simulink model "S250205simul_switch_2023a"  (R2024b)
settings: Solver=FixedStepDiscrete  StartTime=0  StopTime=60  FixedStep=0.01  RelTol=1e-3  AbsTol=1e-6
undefined symbols (not defined in the file or in its folder): a, b, c, d, f, g, switch_logic, VmcRgn_C_C, VmcRgn_J_C, VmcRgn_k_1to2_C, VmcRgn_k_2to3_C, VmcRgn_k_2to6_C, VmcRgn_k_3to4_C, VmcRgn_k_5to2_C, VmcRgn_k_6to2_C, VmcRgn_Kp_C, VmcRgn_L_C, VmcRgn_lf_C, VmcRgn_lr_C, VmcRgn_mass_C, VmcRgn_Mot2Whl_C, VmcRgn_PedDep_thrs_C, VmcRgn_phs2_k_C, VmcRgn_phs2_tq_C, VmcRgn_phs3_tq_C, VmcRgn_phs4_tq_C, VmcRgn_phs5_tq_C, VmcRgn_phs6_tq_C, VmcRgn_r_e_C, VmcRgn_R_whl_C, VmcRgn_SAS_thrs_C, VmcRgn_slip_max_C, VmcRgn_slip_max_gain_F_C, VmcRgn_slip_max_gain_R_C, VmcRgn_sup_tq_C, VmcRgn_t_pred_C, VmcRgn_target_w_acc_C, VmcRgn_tTs, VmcRgn_tTsinMs_C, VmcRgn_Yaw_thrs_C, yaw_flag
libraries: simulink x26, simulink_need_slupdate x1
(part 1 of 3)
settings Model: Creator=jhu  LastModifiedBy=jshan
settings SolverCC: AutoScaleAbsTol=off
settings DataIOCC: SaveFormat=Array  SignalLoggingSaveFormat=ModelDataLogs  ReturnWorkspaceOutputs=off  SignalLoggingName=sigsOut
settings OptimizationCC: BlockReduction=off  BooleanDataType=off  ExpressionDepthLimit=2147483647  LifeSpan=inf
settings DebuggingCC: SaveWithParameterizedLinksMsg=none  UnderspecifiedInitializationDetection=Classic  MergeDetectMultiDrivingBlocksExec=none  SignalResolutionControl=TryResolveAllWithWarning  MultiTaskDSMMsg=warning  MultiTaskCondExecSysMsg=none  FcnCallInpInsideContextMsg=warning  UnconnectedInputMsg=warning  UnconnectedOutputMsg=warning  UnconnectedLineMsg=warning  StateNameClashWarn=warning  SFUnexpectedBacktrackingDiag=warning  SFNoUnconditionalDefaultTransitionDiag=warning  SFExecutionAtInitializationDiag=none  ArithmeticOperatorsInVariantConditions=warning
settings HardwareCC: ProdBitPerPointer=32  ProdBitPerSizeT=32  ProdBitPerPtrDiffT=32  ProdLargestAtomicFloat=None  ProdIntDivRoundTo=Undefined  ProdEndianess=Unspecified  ProdWordSize=32  ProdHWDeviceType=32-bit Generic  TargetUnknown=on
settings ModelReferenceCC: PropagateSignalLabelsOutOfModel=off
settings SFSimCC: SimUseLocalCustomCode=off  CustomCodeUndefinedFunction=UseInterfaceOnly
settings RTWCC: TemplateMakefile=grt_vc.tmf  RTWUseLocalCustomCode=off  GPUComputeCapability=3.5
settings CodeAppCC: StateflowObjectComments=on
settings GRTTargetCC: TargetFcnLib=ansi_tfl_tmw.mat  TargetLangStandard=C89/C90 (ANSI)  CombineOutputUpdateFcns=off  GRTInterface=on
settings ConfigComp: CovMetricSettings=dw  CovSaveCumulativeToWorkspaceVar=on  CovSaveSingleToWorkspaceVar=on  CovExternalEMLEnable=off

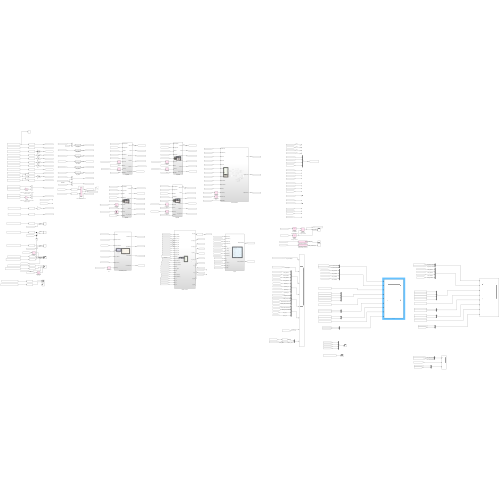
[thumbnail: Simulink's stored preview of the top-level diagram]
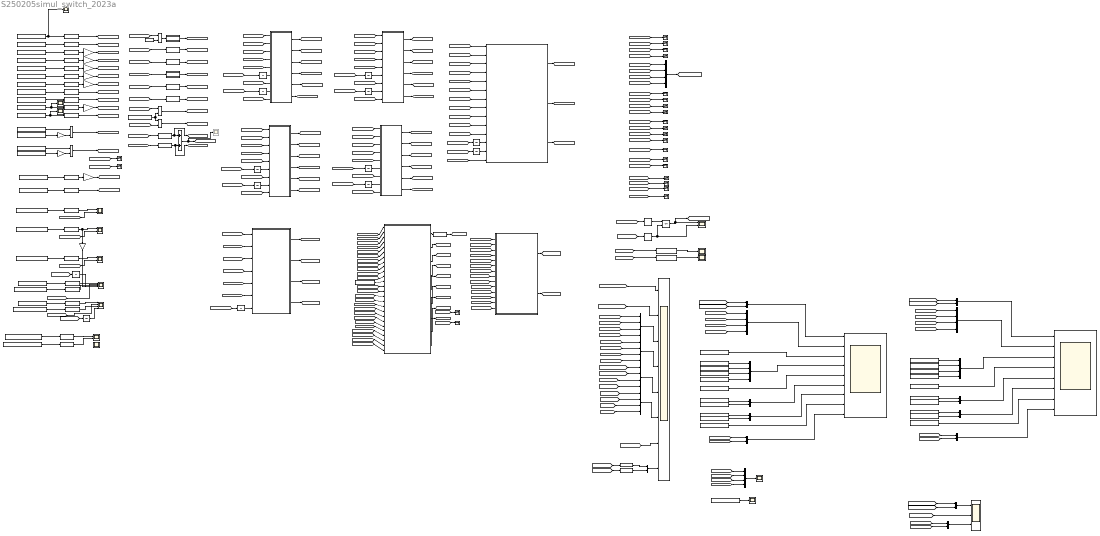
== system S250205simul_switch_2023a ==
  note: VCU_MotTqCmdFrntVal
  note: VCU_MotTqCmdFrntVal
  Add10 : Sum  OutDataTypeStr=fixdt(1,16,2^0,0)  AccumDataTypeStr=single  RndMeth=Round  SaturateOnIntegerOverflow=on  LockScale=on
      settings: AttributesFormatString=OutType: %<OutDataTypeStr>
  Compare To Constant : simulink/Logic and Bit Operations/Compare To Constant  relop=>=  const=2  OutDataTypeStr=boolean
      settings: AttributesFormatString=OutType: %<OutDataTypeStr>
  Compare To Zero : simulink/Logic and Bit Operations/Compare To Zero  relop=~=  OutDataTypeStr=boolean
      settings: AttributesFormatString=OutType: %<OutDataTypeStr>
  Constant : Constant  Value=1/3.6  OutDataTypeStr=single
  Data Type Conversion{,1..13,16..28} (27 alike) : DataTypeConversion  OutDataTypeStr=single  SaturateOnIntegerOverflow=off  RndMeth=Floor
  Data Type Conversion14 : DataTypeConversion  OutDataTypeStr=fixdt(1,16,2^-3,0)  RndMeth=Round  LockScale=on
      settings: AttributesFormatString=OutType: %<OutDataTypeStr>
  Data Type Conversion15 : DataTypeConversion  OutDataTypeStr=fixdt(1,16,2^-3,0)  RndMeth=Round  LockScale=on
      settings: AttributesFormatString=OutType: %<OutDataTypeStr>
  From Workspace : FromWorkspace  VariableName=[t VseSpd_sEstSpdFilt]  SampleTime=-1
  From Workspace1 : FromWorkspace  VariableName=[t IsAcu_dsLongAccl]  SampleTime=-1
  From Workspace10 : FromWorkspace  VariableName=[t IsHal_pcAlgAps]  SampleTime=-1
  From Workspace11 : FromWorkspace  VariableName=[t VCU_StdMotTqFrntVal]  SampleTime=-1
  From Workspace12 : FromWorkspace  VariableName=[t PtMot_pcBItvTqCmdFrnt]  SampleTime=-1
  From Workspace13 : FromWorkspace  VariableName=[t VCU_StdMotTqRearVal]  SampleTime=-1
  From Workspace14 : FromWorkspace  VariableName=[t PtMot_pcBItvTqCmdRear]  SampleTime=-1
  From Workspace15 : FromWorkspace  VariableName=[t IsIeb_dDrvBrkStrk_mm]  SampleTime=-1
  From Workspace16 : FromWorkspace  VariableName=[t VseLat_dradTarYawRate]
  From Workspace17 : FromWorkspace  VariableName=[t Tp_VmcRgn_stSMWUState]  SampleTime=-1
  From Workspace18 : FromWorkspace  VariableName=[t VmcRgn_fSMWUActSta]  SampleTime=-1
  From Workspace19 : FromWorkspace  VariableName=[t VseSpd_rSlipRtFilWhlFl]  SampleTime=-1
  From Workspace2 : FromWorkspace  VariableName=[t IsAcu_daYawRate]  SampleTime=-1
  From Workspace20 : FromWorkspace  VariableName=[t VCU_MotTqCmdFrntVal]  SampleTime=-1
  From Workspace21 : FromWorkspace  VariableName=[t VCU_MotTqCmdRearVal]  SampleTime=-1
  From Workspace22 : FromWorkspace  VariableName=[t VmcRgn_tqSMWUFrntTqCmd]  SampleTime=-1
  From Workspace23 : FromWorkspace  VariableName=[t VmcRgn_tqSMWURearTqCmd]  SampleTime=-1
  From Workspace24 : FromWorkspace  VariableName=[t Tp_VmcRgn_tqSMWU_TbMaxFrnt]  SampleTime=-1
  From Workspace25 : FromWorkspace  VariableName=[t Tp_VmcRgn_tqSMWU_TbMaxRear]  SampleTime=-1
  From Workspace26 : FromWorkspace  VariableName=[t Tp_VmcRgn_stSMWUSlipPhaseFL]
  From Workspace27 : FromWorkspace  VariableName=[t Tp_VmcRgn_stSMWUSlipPhaseFR]
  From Workspace28 : FromWorkspace  VariableName=[t Tp_VmcRgn_stSMWUSlipPhaseRL]
  From Workspace29 : FromWorkspace  VariableName=[t Tp_VmcRgn_stSMWUSlipPhaseRR]
  From Workspace3 : FromWorkspace  VariableName=[t IsIeb_sWhlSpdFl]  SampleTime=-1
  From Workspace30 : FromWorkspace  VariableName=[t Tp_VmcRgn_stSMWUState]
  From Workspace31 : FromWorkspace  VariableName=[t VmcRgn_fSMWUActSta]
  From Workspace32 : FromWorkspace  VariableName=[t Tp_VmcRgn_fSMWUYawFlag]
  From Workspace33 : FromWorkspace  VariableName=[t Tp_VmcRgn_tqSMWU_TbMaxFrnt]
  From Workspace34 : FromWorkspace  VariableName=[t Tp_VmcRgn_tqSMWU_TbMaxRear]
  From Workspace35 : FromWorkspace  VariableName=[t IsHal_pcAlgAps]  SampleTime=-1
  From Workspace36 : FromWorkspace  VariableName=[t IsSas_aStrWhlAngle]  SampleTime=-1
  From Workspace37 : FromWorkspace  VariableName=[t Tp_VmcRgn_stSMWUSlipPhaseFL]
  From Workspace38 : FromWorkspace  VariableName=[t Tp_VmcRgn_stSMWUSlipPhaseFR]
  From Workspace39 : FromWorkspace  VariableName=[t Tp_VmcRgn_stSMWUSlipPhaseRL]
  From Workspace4 : FromWorkspace  VariableName=[t IsIeb_sWhlSpdFr]  SampleTime=-1
  From Workspace40 : FromWorkspace  VariableName=[t Tp_VmcRgn_stSMWUSlipPhaseRR]
  From Workspace41 : FromWorkspace  VariableName=[t Tp_VmcRgn_stSMWUState]
  From Workspace42 : FromWorkspace  VariableName=[t VmcRgn_fSMWUActSta]
  From Workspace43 : FromWorkspace  VariableName=[t Tp_VmcRgn_fSMWUYawFlag]
  From Workspace44 : FromWorkspace  VariableName=[t Tp_VmcRgn_tqSMWU_TbMaxFrnt]
  From Workspace45 : FromWorkspace  VariableName=[t Tp_VmcRgn_tqSMWU_TbMaxRear]
  From Workspace46 : FromWorkspace  VariableName=[t IsHal_pcAlgAps]  SampleTime=-1
  From Workspace47 : FromWorkspace  VariableName=[t IsSas_aStrWhlAngle]  SampleTime=-1
  From Workspace5 : FromWorkspace  VariableName=[t IsIeb_sWhlSpdRl]  SampleTime=-1
  From Workspace6 : FromWorkspace  VariableName=[t IsIeb_sWhlSpdRr]  SampleTime=-1
  From Workspace7 : FromWorkspace  VariableName=[t VCU_MotTqCmdFrntVal]  SampleTime=-1
  From Workspace8 : FromWorkspace  VariableName=[t VCU_MotTqCmdRearVal]  SampleTime=-1
  From Workspace9 : FromWorkspace  VariableName=[t IsSas_aStrWhlAngle]  SampleTime=-1
  Gain : Gain  Gain=-50
  Gain1 : Gain  Gain=-1
  Gain{7..10} (4 alike) : Gain  Gain=1/3.6
  Gain3 : Gain  Gain=0.01  ParamDataTypeStr=Inherit: Inherit from 'Gain'  OutDataTypeStr=single  RndMeth=Round  SaturateOnIntegerOverflow=on
      settings: AttributesFormatString=ParamType: %<ParamDataTypeStr>\nOutType: %<OutDataTypeStr>
  Gain4 : Gain  Gain=0.01  ParamDataTypeStr=Inherit: Inherit from 'Gain'  OutDataTypeStr=single  RndMeth=Round  SaturateOnIntegerOverflow=on
      settings: AttributesFormatString=ParamType: %<ParamDataTypeStr>\nOutType: %<OutDataTypeStr>
  Gain5 : Gain  Gain=pi/180
  Gain6 : Gain  Gain=pi/180
  LPF_5Hz : Subsystem
  LPF_5Hz1 : Subsystem
  LPF_5Hz2 : Subsystem
  LPF_5Hz3 : Subsystem
  LPF_5Hz4 : Subsystem
  LPF_5Hz5 : Subsystem
  Logical Operator31 : Logic  Operator=OR  OutDataTypeStr=boolean
      settings: AttributesFormatString=OutType: %<OutDataTypeStr>
  Mot2Whl : Constant  Value=VmcRgn_Mot2Whl_C  OutDataTypeStr=single
  Mot2Whl1 : Constant  Value=VmcRgn_Mot2Whl_C
  Mux{,1..2,4,6..8,15..16,18} (10 alike) : Mux
  Mux{3,5,9..14,17,19..20} (11 alike) : Mux  Inputs=2
  Product{3..4,10..12} (5 alike) : Product
  "Regen, Tb_max1" : Subsystem
  Scope{,6..8,11} (5 alike) : Scope  NumInputPorts=2
  Scope{1..2,12..16,18} (8 alike) : Scope
  Scope10 : Scope  NumInputPorts=4
  Scope17 : Scope  NumInputPorts=8
  Scope19 : Scope  NumInputPorts=3
  Scope3 : Scope  NumInputPorts=8
  Scope4 : Scope  NumInputPorts=9
  Scope5 : Scope  Commented=on
  Scope9 : Scope  NumInputPorts=5
  Slip Control State1 : Subsystem
  SlipCtrlFL : Subsystem
  SlipCtrlFR : Subsystem
  SlipCtrlRL : Subsystem
  SlipCtrlRR : Subsystem
  Terminator{,1..3,8..26} (23 alike) : Terminator
  Torque : Subsystem
  Unit Delay{1..11,21..22} (13 alike) : UnitDelay  SampleTime=-1  HasFrameUpgradeWarning=on  mask(Customized Unit Delay){}
      settings: AttributesFormatString=IC: %<X0>
  Yaw Stability Control1 : Subsystem
  wires:
  Data Type Conversion15/1 -> Scope2/1  "SMWU_RearMtTqCmd"
  Data Type Conversion14/1 -> Scope1/1  "SMWU_FrntMtTqCmd"
  [MotTqCmdRearVal] -> Data Type Conversion15/1
  [MotTqCmdFrntVal] -> Data Type Conversion14/1
  Logical Operator31/1 -> [SMWU_ActSta], Scope/1  "SMWU_ActSta"
  Compare To Zero/1 -> Scope/2, Logical Operator31/2
  Compare To Constant/1 -> Logical Operator31/1
  [yaw_flag] -> Compare To Zero/1
  [State] -> Compare To Constant/1
  [VCU_BInvRearNmVal] -> Terminator24/1
  [VCU_BInvFrntNmVal] -> Terminator23/1
  Gain10/1 -> [WHL_SpdRRVal]
  Gain9/1 -> [WHL_SpdRLVal]
  Gain8/1 -> [WHL_SpdFRVal]
  Gain7/1 -> [WHL_SpdFLVal]
  Add10/1 -> Scope5/1, [RegenCmdTq]
  Data Type Conversion12/1 -> Add10/1, [MotCoastFrntTq]
  Data Type Conversion13/1 -> Add10/2, [MotCoastRearTq]
  Unit Delay10/1 -> Slip Control State1/13(RearCmdTq)
  Unit Delay9/1 -> Slip Control State1/12(FrntCmdTq)
  [MotTqCmdRearVal] -> Unit Delay10/1
  [MotTqCmdFrntVal] -> Unit Delay9/1
  Unit Delay8/1 -> SlipCtrlRR/8(YawFlag)
  Unit Delay7/1 -> SlipCtrlRR/6(TqCtrlVal)
  Unit Delay6/1 -> SlipCtrlRL/8(YawFlag)
  Unit Delay5/1 -> SlipCtrlRL/6(TqCtrlVal)
  Unit Delay3/1 -> SlipCtrlFR/8(YawFlag)
  Unit Delay2/1 -> SlipCtrlFR/6(TqCtrlVal)
  Unit Delay1/1 -> SlipCtrlFL/8(YawFlag)
  Unit Delay4/1 -> SlipCtrlFL/6(TqCtrlVal)
  Gain6/1 -> [SAS_AnglVal]
  Product11/1 -> [VCU_BInvRearNmVal]
  Product3/1 -> [VCU_BInvFrntNmVal]
  Gain4/1 -> Product11/2
  Gain3/1 -> Product3/2
  From Workspace14/1 -> Gain4/1
  From Workspace13/1 -> Product11/1
  From Workspace12/1 -> Gain3/1
  From Workspace11/1 -> Product3/1
  [VCU_BInvRearNmVal] -> Data Type Conversion13/1
  [VCU_BInvFrntNmVal] -> Data Type Conversion12/1
  [MotTqCmdFrntVal] -> Unit Delay2/1
  [MotTqCmdRearVal] -> Unit Delay7/1
  [MotTqCmdRearVal] -> Unit Delay5/1
  [MotTqCmdRearVal] -> "Regen, Tb_max1"/16(MotTqCmdRearVal)
  [yaw_flag] -> Unit Delay8/1
  [yaw_flag] -> Unit Delay3/1
  [yaw_flag] -> Unit Delay1/1
  [MotTqCmdFrntVal] -> Unit Delay4/1
  From Workspace10/1 -> Scope16/1, Data Type Conversion10/1
  From Workspace9/1 -> Scope15/1, Data Type Conversion11/1
  From Workspace/1 -> Scope14/1, Data Type Conversion/1
  From Workspace1/1 -> Data Type Conversion2/1
  From Workspace3/1 -> Data Type Conversion4/1
  From Workspace4/1 -> Data Type Conversion5/1
  From Workspace5/1 -> Data Type Conversion6/1
  From Workspace6/1 -> Data Type Conversion7/1
  From Workspace7/1 -> Data Type Conversion8/1
  From Workspace8/1 -> Data Type Conversion9/1
  [yaw_flag] -> Unit Delay6/1
  [SlipPhase_FR] -> Slip Control State1/8(SlipPhaseFR)
  Slip Control State1/3(SlipCtrlRearTq) -> [SlipCtrlRearTq]
  Slip Control State1/1(State) -> [State]
  LPF_5Hz3/1(Out1) -> [WHL_SpdFRFlt]  "filtered"
  [VehicleSpdFlt] -> SlipCtrlFL/1(VehicleSpdFlt)
  [WHL_SpdRRFlt] -> SlipCtrlRR/4(WhlSpdFlt)
  [IMU_LongAccelFlt] -> SlipCtrlRL/2(LongAccelFlt)
  [MotCoastRearTq] -> Slip Control State1/2(CoastRearTq)
  [WhlTqFrntVal] -> SlipCtrlFR/7(WhlTq)
  Slip Control State1/2(SlipCtrlFrntTq) -> [SlipCtrlFrntTq]
  [SlipCtrlTq_FL] -> Slip Control State1/3(TqCtrlFL)
  [VehicleSpdFlt] -> SlipCtrlRL/1(VehicleSpdFlt)
  [SlipPhase_FL] -> Slip Control State1/7(SlipPhaseFL)
  [MotCoastFrntTq] -> Slip Control State1/1(CoastFrntTq)
  SlipCtrlRL/4(SlipPhase) -> [SlipPhase_RL]
  [SlipCtrlTq_FR] -> Slip Control State1/4(TqCtrlFR)
  [WHL_SpdFLFlt] -> SlipCtrlFL/4(WhlSpdFlt)
  [MotCoastRearTq] -> SlipCtrlRL/5(CoastTq)
  [SlipPhase_RR] -> Slip Control State1/10(SlipPhaseRR)
  [SlipCtrlTq_RL] -> Slip Control State1/5(TqCtrlRL)
  [SlipPhase_RL] -> Slip Control State1/9(SlipPhaseRL)
  SlipCtrlRL/5(SlipCtrlTq) -> [SlipCtrlTq_RL]
  [VCU_AccPedDepVal] -> Slip Control State1/11(PedDep)
  [WHL_SpdRLFlt] -> SlipCtrlRL/4(WhlSpdFlt)
  SlipCtrlRR/4(SlipPhase) -> [SlipPhase_RR]
  SlipCtrlRR/2(SlipVal) -> [SlipVal_RR]
  SlipCtrlRL/2(SlipVal) -> [SlipVal_RL]
  [VCU_MotTqCmdRearVal] -> Product4/2
  Mot2Whl/1 -> Product4/1, Product12/2
  SlipCtrlFR/1(TireForce) -> [TireForce_FR]
  [WhlTqRearVal] -> SlipCtrlRR/7(WhlTq)
  SlipCtrlRR/3(SlipPredVal) -> [SlipPredVal_RR]
  [VCU_AccPedDepVal] -> SlipCtrlRR/9(PedDep)
  [SlipCtrlTq_RR] -> Slip Control State1/6(TqCtrlRR)
  SlipCtrlRR/5(SlipCtrlTq) -> [SlipCtrlTq_RR]
  SlipCtrlRL/3(SlipPredVal) -> [SlipPredVal_RL]
  [VehicleSpdFlt] -> SlipCtrlFR/1(VehicleSpdFlt)
  [VehicleSpdFlt] -> SlipCtrlRR/1(VehicleSpdFlt)
  SlipCtrlFR/3(SlipPredVal) -> [SlipPredVal_FR]
  [WhlTqRearVal] -> SlipCtrlRL/7(WhlTq)
  SlipCtrlFR/5(SlipCtrlTq) -> [SlipCtrlTq_FR]
  [VCU_AccPedDepVal] -> SlipCtrlFR/9(PedDep)
  [VCU_AccPedDepVal] -> SlipCtrlRL/9(PedDep)
  [MotCoastRearTq] -> SlipCtrlRR/5(CoastTq)
  SlipCtrlRL/1(TireForce) -> [TireForce_RL]
  SlipCtrlFL/4(SlipPhase) -> [SlipPhase_FL]
  [WhlTqFrntVal] -> SlipCtrlFL/7(WhlTq)
  [MotCoastFrntTq] -> SlipCtrlFR/5(CoastTq)
  [IMU_LongAccelFlt] -> SlipCtrlFL/2(LongAccelFlt)
  [IMU_LongAccelFlt] -> SlipCtrlFR/2(LongAccelFlt)
  SlipCtrlFL/3(SlipPredVal) -> [SlipPredVal_FL]
  [WHL_SpdRLVal] -> LPF_5Hz4/1(In1)
  SlipCtrlFL/1(TireForce) -> [TireForce_FL]
  LPF_5Hz5/1(Out1) -> [WHL_SpdRRFlt]  "filtered"
  [VCU_AccPedDepVal] -> SlipCtrlFL/9(PedDep)
  SlipCtrlRR/1(TireForce) -> [TireForce_RR]
  SlipCtrlFL/5(SlipCtrlTq) -> [SlipCtrlTq_FL]
  SlipCtrlFR/2(SlipVal) -> [SlipVal_FR]
  [IMU_LongAccelVal] -> LPF_5Hz1/1(In1)
  LPF_5Hz2/1(Out1) -> [WHL_SpdFLFlt]  "filtered"
  [WHL_SpdFLVal] -> LPF_5Hz2/1(In1)
  [WHL_SpdFRVal] -> LPF_5Hz3/1(In1)
  Product10/1 -> LPF_5Hz/1(In1)
  LPF_5Hz4/1(Out1) -> [WHL_SpdRLFlt]  "filtered"
  SlipCtrlFR/4(SlipPhase) -> [SlipPhase_FR]
  Constant/1 -> Product10/2
  [WHL_SpdRRVal] -> LPF_5Hz5/1(In1)
  Product12/1 -> [WhlTqFrntVal]
  [VCU_MotTqCmdFrntVal] -> Product12/1
  SlipCtrlFL/2(SlipVal) -> [SlipVal_FL]
  [WHL_SpdFRFlt] -> SlipCtrlFR/4(WhlSpdFlt)
  [VehicleSpdVal] -> Product10/1
  LPF_5Hz1/1(Out1) -> [IMU_LongAccelFlt]  "filtered"
  [MotCoastFrntTq] -> SlipCtrlFL/5(CoastTq)
  Product4/1 -> [WhlTqRearVal]
  [IMU_LongAccelFlt] -> SlipCtrlRR/2(LongAccelFlt)
  [Tb_max_Frnt] -> Torque/6(Tb_max_F)
  [H_R] -> Torque/11(H_R)
  [YawCtrlFrntTq] -> Torque/3(YawCtrlFrntTq)
  [IMU_YawRtVal] -> "Regen, Tb_max1"/2(IMU_YawRtVal)
  "Regen, Tb_max1"/5(Tb_max_R) -> [Tb_max_Rear]
  [DesYawRtVal] -> "Regen, Tb_max1"/1(DesYawRtVal)
  [YawCtrlRearTq] -> Torque/4(YawCtrlRearTq)
  [MotCoastFrntTq] -> Torque/8(CoastFrntTq)
  [MotCoastRearTq] -> Torque/9(CoastRearTq)
  Torque/2(MotTqCmdRearVal) -> [MotTqCmdRearVal]
  "Regen, Tb_max1"/4(Tb_max_F) -> [Tb_max_Frnt]
  [Tr_regen_2] -> Torque/12(Tr_regen_2)
  [H_F] -> Torque/10(H_F)
  "Regen, Tb_max1"/9(Tr_regen) -> [Tr_regen]
  [Tb_max_Rear] -> Torque/7(Tb_max_R)
  "Regen, Tb_max1"/2(Tr_regen_2) -> [Tr_regen_2]
  "Regen, Tb_max1"/7(H_R) -> [H_R]
  "Regen, Tb_max1"/8(Tf_regen) -> [Tf_regen]
  "Regen, Tb_max1"/1(yaw_flag) -> Data Type Conversion18/1
  [Tf_regen_3] -> Torque/13(Tf_regen_3)
  Torque/1(MotTqCmdFrntVal) -> [MotTqCmdFrntVal]
  "Regen, Tb_max1"/3(Tf_regen_3) -> [Tf_regen_3]
  "Regen, Tb_max1"/6(H_F) -> [H_F]
  [TireForce_RL] -> "Regen, Tb_max1"/6(TireForce_RL)
  [SlipPredVal_RL] -> "Regen, Tb_max1"/10(slip_pred_RL)
  Mot2Whl1/1 -> "Regen, Tb_max1"/12(mot2whl)
  [SlipCtrlRearTq] -> Torque/2(SlipCtrlRearTq)
  [State] -> Torque/5(State)
  [TireForce_RR] -> "Regen, Tb_max1"/7(TireForce_RR)
  [TireForce_FR] -> "Regen, Tb_max1"/5(TireForce_FR)
  [TireForce_FL] -> "Regen, Tb_max1"/4(TireForce_FL)
  [SlipPredVal_FL] -> "Regen, Tb_max1"/8(slip_pred_FL)
  [SlipPredVal_FR] -> "Regen, Tb_max1"/9(slip_pred_FR)
  [SlipPredVal_RR] -> "Regen, Tb_max1"/11(slip_pred_RR)
  [RegenCmdTq] -> "Regen, Tb_max1"/3(regen_cmd_tq)
  [SlipCtrlFrntTq] -> "Regen, Tb_max1"/13(SlipCtrlFrntTq)
  [SlipCtrlRearTq] -> "Regen, Tb_max1"/14(SlipCtrlRearTq)
  [MotTqCmdFrntVal] -> "Regen, Tb_max1"/15(MotTqCmdFrntVal)
  [yaw_flag] -> Torque/14(yaw_flag)
  Yaw Stability Control1/3(DesYawRtVal) -> [DesYawRtVal]
  Yaw Stability Control1/1(YawCtrlFrntTq) -> [YawCtrlFrntTq]
  Yaw Stability Control1/2(YawCtrlRearTq) -> [YawCtrlRearTq]
  [State] -> Yaw Stability Control1/4(State)
  [MotTqCmdFrntVal] -> Yaw Stability Control1/2(MotTqCmdFrntVal)
  [MotTqCmdRearVal] -> Yaw Stability Control1/3(MotTqCmdRearVal)
  Data Type Conversion2/1 -> [IMU_LongAccelVal]
  Data Type Conversion10/1 -> [VCU_AccPedDepVal]
  Data Type Conversion8/1 -> [VCU_MotTqCmdFrntVal]
  Data Type Conversion/1 -> [VehicleSpdVal]
  Data Type Conversion7/1 -> Gain10/1
  Data Type Conversion4/1 -> Gain7/1
  Data Type Conversion9/1 -> [VCU_MotTqCmdRearVal]
  Data Type Conversion11/1 -> Gain6/1
  Data Type Conversion5/1 -> Gain8/1
  Data Type Conversion3/1 -> Gain5/1
  Yaw Stability Control1/4(CorrYawMmtVal) -> [CorrYawMmtVal]
  [SlipCtrlFrntTq] -> Torque/1(SlipCtrlFrntTq)
  Data Type Conversion6/1 -> Gain9/1
  [WHL_SpdFLVal] -> SlipCtrlFL/3(WhlSpd)
  [WHL_SpdRLVal] -> SlipCtrlRL/3(WhlSpd)
  [WHL_SpdRRVal] -> SlipCtrlRR/3(WhlSpd)
  [WHL_SpdFRVal] -> SlipCtrlFR/3(WhlSpd)
  [CorrYawMmtVal] -> Terminator22/1
  [DesYawRtVal] -> Terminator21/1
  [YawCtrlRearTq] -> Terminator20/1
  [YawCtrlFrntTq] -> Terminator19/1
  [SlipVal_RL] -> Mux18/3
  [TireForce_RL] -> Terminator2/1
  [SlipPhase_FR] -> Terminator13/1
  [SlipPredVal_RL] -> Terminator10/1
  [SlipVal_FR] -> Mux18/2
  [SlipVal_RR] -> Mux18/4
  [TireForce_FR] -> Terminator1/1
  [SlipPhase_FL] -> Terminator12/1
  [SlipVal_FL] -> Mux18/1
  [SlipPredVal_RR] -> Terminator11/1
  [TireForce_FL] -> Terminator/1
  [SlipCtrlRearTq] -> Terminator18/1
  [SlipPhase_RL] -> Terminator14/1
  [State] -> Terminator16/1
  [SlipPredVal_FR] -> Terminator9/1
  [SlipPhase_RR] -> Terminator15/1
  [TireForce_RR] -> Terminator3/1
  [SlipCtrlFrntTq] -> Terminator17/1
  [SlipPredVal_FL] -> Terminator8/1
  [VCU_MotTqCmdFrntVal] -> Mux/1  "VCU_MotTqCmdFrntVal"
  [VCU_MotTqCmdRearVal] -> Mux/2  "VCU_MotTqCmdRearVal"
  [MotTqCmdFrntVal] -> Mux/3  "SMWU_MotTqCmdFrntVal"
  [MotTqCmdRearVal] -> Mux/4  "SMWU_MotTqCmdRearVal"
  Mux/1 -> Scope3/5
  Mux1/1 -> Scope3/6
  [MotTqCmdRearVal] -> Mux1/2  "SMWU_MotTqCmdRearVal"
  [MotTqCmdFrntVal] -> Mux1/1  "SMWU_MotTqCmdFrntVal"
  [Tb_max_Frnt] -> Mux1/3  "Tb_max_F"
  [Tb_max_Rear] -> Mux1/4  "Tb_max_R"
  [SlipPhase_FL] -> Mux2/1  "SlipPhase_FL"
  [SlipPhase_FR] -> Mux2/2  "SlipPhase_FR"
  [SlipPhase_RL] -> Mux2/3  "SlipPhase_RL"
  [SlipPhase_RR] -> Mux2/4  "SlipPhase_RR"
  [VCU_AccPedDepVal] -> Scope3/1  "VCU_AccPedDepVal"
  [SAS_AnglVal] -> Scope3/2  "SAS_AnglVal"
  [State] -> Scope3/7  "ControlState"
  Mux2/1 -> Scope3/4
  [SMWU_ActSta] -> Data Type Conversion19/1  "SMWU_ActSta"
  Mux3/1 -> Scope3/8
  Mux4/1 -> Scope3/3
  [WHL_SpdRLVal] -> Mux4/3  "WHL_SpdRLVal"
  [WHL_SpdRRVal] -> Mux4/4  "WHL_SpdRRVal"
  [WHL_SpdFRVal] -> Mux4/2  "WHL_SpdFRVal"
  [WHL_SpdFLVal] -> Mux4/1  "WHL_SpdFLVal"
  [yaw_flag] -> Data Type Conversion1/1
  [VCU_AccPedDepVal] -> "Regen, Tb_max1"/17(PedDep)
  [SAS_AnglVal] -> "Regen, Tb_max1"/18(SAS_AnglVal)
  [VCU_BrkPedDepVal] -> "Regen, Tb_max1"/19(BrkPed)
  From Workspace2/1 -> Data Type Conversion3/1
  Gain5/1 -> [IMU_YawRtVal]
  Data Type Conversion16/1 -> Gain1/1
  From Workspace15/1 -> Data Type Conversion17/1
  Gain1/1 -> [Des_YawRtVal_HMC]
  [Des_YawRtVal_HMC] -> Yaw Stability Control1/5(Des_YawRtVal)
  [IMU_YawRtVal] -> Yaw Stability Control1/1(YawRtVal)
  [State] -> "Regen, Tb_max1"/20(State)
  Data Type Conversion17/1 -> [VCU_BrkPedDepVal]
  From Workspace16/1 -> Data Type Conversion16/1
  [VCU_BrkPedDepVal] -> Slip Control State1/14(BrkPedDep)
  [MotCoastFrntTq] -> "Regen, Tb_max1"/21(MotCoastFrntTq)
  [MotCoastRearTq] -> "Regen, Tb_max1"/22(MotCoastRearTq)
  Data Type Conversion1/1 -> Mux3/1  "yaw_flag"
  Data Type Conversion19/1 -> Mux3/2  "SMWU_ActSta"
  From Workspace17/1 -> Data Type Conversion20/1
  Data Type Conversion20/1 -> Scope6/1  "realCar"
  [State] -> Scope6/2  "sim"
  [SMWU_ActSta] -> Scope7/2  "sim"
  Data Type Conversion21/1 -> Gain/1, Scope7/1  "realCar"
  From Workspace18/1 -> Data Type Conversion21/1
  [SlipVal_FL] -> Scope8/2  "sim"
  Data Type Conversion22/1 -> Scope8/1  "realCar"
  From Workspace19/1 -> Data Type Conversion22/1
  LPF_5Hz/1(Out1) -> [VehicleSpdFlt]  "filtered"
  From Workspace21/1 -> Data Type Conversion24/1
  From Workspace20/1 -> Data Type Conversion23/1
  Data Type Conversion23/1 -> Scope9/1  "Car"
  Data Type Conversion24/1 -> Scope10/1
  [MotTqCmdFrntVal] -> Unit Delay21/1
  [MotTqCmdRearVal] -> Unit Delay22/1
  Unit Delay22/1 -> Scope10/4
  Unit Delay21/1 -> Scope9/4  "Sim"
  From Workspace22/1 -> Data Type Conversion25/1
  From Workspace23/1 -> Data Type Conversion26/1
  Data Type Conversion26/1 -> Scope10/3
  Data Type Conversion25/1 -> Scope9/3  "Ctrl"
  [MotCoastFrntTq] -> Scope9/2  "Blnv"
  Gain/1 -> Scope9/5
  [Tf_regen] -> Terminator25/1
  [Tr_regen] -> Terminator26/1
  Data Type Conversion18/1 -> [yaw_flag]
  [MotCoastRearTq] -> Scope10/2  "Blnv"
  From Workspace24/1 -> Data Type Conversion27/1
  Data Type Conversion27/1 -> Scope11/1
  From Workspace25/1 -> Data Type Conversion28/1
  Data Type Conversion28/1 -> Scope11/2
  SlipCtrlRL/6(Tb_max_Hold) -> [H_RL]
  SlipCtrlFL/6(Tb_max_Hold) -> [H_FL]
  SlipCtrlFR/6(Tb_max_Hold) -> [H_FR]
  SlipCtrlRR/6(Tb_max_Hold) -> [H_RR]
  [H_FL] -> "Regen, Tb_max1"/23(H_FL)
  [H_FR] -> "Regen, Tb_max1"/24(H_FR)
  [H_RL] -> "Regen, Tb_max1"/25(H_RL)
  [H_RR] -> "Regen, Tb_max1"/26(H_RR)
  From Workspace29/1 -> Mux8/4
  From Workspace33/1 -> Mux10/1
  Mux8/1 -> Scope4/4
  From Workspace26/1 -> Mux8/1
  Mux11/1 -> Scope4/9
  From Workspace28/1 -> Mux8/3
  From Workspace27/1 -> Mux8/2
  From Workspace30/1 -> Scope4/5
  From Workspace35/1 -> Scope4/8
  From Workspace31/1 -> Mux9/1
  Mux5/1 -> Scope4/1
  From Workspace34/1 -> Mux10/2
  Mux9/1 -> Scope4/6
  [IMU_YawRtVal] -> Mux11/2
  [VCU_MotTqCmdRearVal] -> Mux5/2  "VCU_MotTqCmdRearVal"
  From Workspace32/1 -> Mux9/2
  [VCU_MotTqCmdFrntVal] -> Mux5/1  "VCU_MotTqCmdFrntVal"
  Mux10/1 -> Scope4/7
  [Des_YawRtVal_HMC] -> Mux11/1
  [RegenCmdTq] -> Yaw Stability Control1/6(RegenCmdTq)
  [WHL_SpdFLVal] -> Mux6/1  "WHL_SpdFLVal"
  [WHL_SpdRLVal] -> Mux6/3  "WHL_SpdRLVal"
  Mux6/1 -> Scope4/2
  [WHL_SpdFRVal] -> Mux6/2  "WHL_SpdFRVal"
  [WHL_SpdRRVal] -> Mux6/4  "WHL_SpdRRVal"
  [SlipVal_RL] -> Mux7/3
  [SlipVal_FL] -> Mux7/1
  [SlipVal_FR] -> Mux7/2
  [SlipVal_RR] -> Mux7/4
  Mux7/1 -> Scope13/1
  From Workspace36/1 -> Scope4/3
  [WHL_SpdRRVal] -> Mux15/4  "WHL_SpdRRVal"
  [WHL_SpdFRVal] -> Mux15/2  "WHL_SpdFRVal"
  [WHL_SpdRLVal] -> Mux15/3  "WHL_SpdRLVal"
  Mux15/1 -> Scope17/2
  [WHL_SpdFLVal] -> Mux15/1  "WHL_SpdFLVal"
  From Workspace37/1 -> Mux16/1
  From Workspace43/1 -> Mux17/2
  From Workspace46/1 -> Scope17/7
  From Workspace42/1 -> Mux17/1
  [Des_YawRtVal_HMC] -> Mux13/1
  From Workspace45/1 -> Mux12/2
  [VCU_MotTqCmdRearVal] -> Mux14/2  "VCU_MotTqCmdRearVal"
  From Workspace39/1 -> Mux16/3
  From Workspace44/1 -> Mux12/1
  [IMU_YawRtVal] -> Mux13/2
  From Workspace41/1 -> Scope17/4
  [VCU_MotTqCmdFrntVal] -> Mux14/1  "VCU_MotTqCmdFrntVal"
  Mux17/1 -> Scope17/5
  From Workspace40/1 -> Mux16/4
  Mux12/1 -> Scope17/6
  Mux16/1 -> Scope17/3
  From Workspace38/1 -> Mux16/2
  Mux14/1 -> Scope17/1
  Mux13/1 -> Scope17/8
  From Workspace47/1 -> Scope18/1
  [yaw_flag] -> Unit Delay11/1
  Unit Delay11/1 -> Yaw Stability Control1/7(Yaw Flag)
  Mux18/1 -> [SlipRatio]
  [VCU_MotTqCmdRearVal] -> Mux19/2  "VCU_MotTqCmdRearVal"
  [VCU_MotTqCmdFrntVal] -> Mux19/1  "VCU_MotTqCmdFrntVal"
  [Des_YawRtVal_HMC] -> Mux20/1
  [IMU_YawRtVal] -> Mux20/2
  Mux19/1 -> Scope19/1
  [SlipRatio] -> Scope19/2
  Mux20/1 -> Scope19/3

== system S250205simul_switch_2023a/LPF_5Hz ==
  In1 : Inport
  Add : Sum  Inputs=+-
  Add1 : Sum
  Delay One Step : Delay  DelayLength=1
  Gain : Gain  Gain=5*2*pi*VmcRgn_tTs/(1+5*2*pi*VmcRgn_tTs)
  Out1 : Outport
  wires:
  In1/1 -> Add/1
  Add/1 -> Gain/1
  Gain/1 -> Add1/1
  Add1/1 -> Delay One Step/1, Out1/1
  Delay One Step/1 -> Add/2, Add1/2

== system S250205simul_switch_2023a/LPF_5Hz1 ==
  In1 : Inport
  Add : Sum  Inputs=+-
  Add1 : Sum
  Delay One Step : Delay  DelayLength=1
  Gain : Gain  Gain=5*2*pi*VmcRgn_tTs/(1+5*2*pi*VmcRgn_tTs)
  Out1 : Outport
  wires:
  Delay One Step/1 -> Add1/2, Add/2
  Add1/1 -> Out1/1, Delay One Step/1
  Gain/1 -> Add1/1
  Add/1 -> Gain/1
  In1/1 -> Add/1

== system S250205simul_switch_2023a/LPF_5Hz2 ==
  In1 : Inport
  Add : Sum  Inputs=+-
  Add1 : Sum
  Delay One Step : Delay  DelayLength=1
  Gain : Gain  Gain=5*2*pi*VmcRgn_tTs/(1+5*2*pi*VmcRgn_tTs)
  Out1 : Outport
  wires:
  In1/1 -> Add/1
  Add/1 -> Gain/1
  Gain/1 -> Add1/1
  Add1/1 -> Delay One Step/1, Out1/1
  Delay One Step/1 -> Add/2, Add1/2

== system S250205simul_switch_2023a/LPF_5Hz3 ==
  In1 : Inport
  Add : Sum  Inputs=+-
  Add1 : Sum
  Delay One Step : Delay  DelayLength=1
  Gain : Gain  Gain=5*2*pi*VmcRgn_tTs/(1+5*2*pi*VmcRgn_tTs)
  Out1 : Outport
  wires:
  Delay One Step/1 -> Add1/2, Add/2
  Add1/1 -> Out1/1, Delay One Step/1
  Gain/1 -> Add1/1
  Add/1 -> Gain/1
  In1/1 -> Add/1

== system S250205simul_switch_2023a/LPF_5Hz4 ==
  In1 : Inport
  Add : Sum  Inputs=+-
  Add1 : Sum
  Delay One Step : Delay  DelayLength=1
  Gain : Gain  Gain=5*2*pi*VmcRgn_tTs/(1+5*2*pi*VmcRgn_tTs)
  Out1 : Outport
  wires:
  In1/1 -> Add/1
  Add/1 -> Gain/1
  Gain/1 -> Add1/1
  Add1/1 -> Delay One Step/1, Out1/1
  Delay One Step/1 -> Add/2, Add1/2

== system S250205simul_switch_2023a/LPF_5Hz5 ==
  In1 : Inport
  Add : Sum  Inputs=+-
  Add1 : Sum
  Delay One Step : Delay  DelayLength=1
  Gain : Gain  Gain=5*2*pi*VmcRgn_tTs/(1+5*2*pi*VmcRgn_tTs)
  Out1 : Outport
  wires:
  Delay One Step/1 -> Add1/2, Add/2
  Add1/1 -> Out1/1, Delay One Step/1
  Gain/1 -> Add1/1
  Add/1 -> Gain/1
  In1/1 -> Add/1

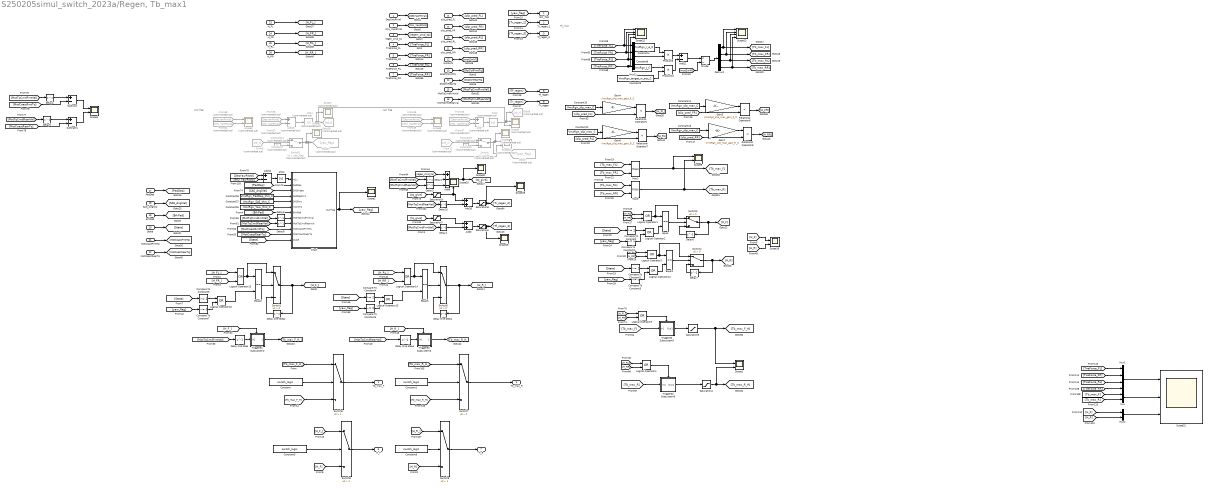
== system S250205simul_switch_2023a/Regen, Tb_max1 ==
  note: Tb_max
  note: yaw flag
  note: yaw flag
  DesYawRtVal : Inport
  IMU_YawRtVal : Inport  Port=2
  regen_cmd_tq : Inport  Port=3
  TireForce_FL : Inport  Port=4
  TireForce_FR : Inport  Port=5
  TireForce_RL : Inport  Port=6
  TireForce_RR : Inport  Port=7
  slip_pred_FL : Inport  Port=8
  slip_pred_FR : Inport  Port=9
  slip_pred_RL : Inport  Port=10
  slip_pred_RR : Inport  Port=11
  mot2whl : Inport  Port=12
  SlipCtrlFrntTq : Inport  Port=13
  SlipCtrlRearTq : Inport  Port=14
  MotTqCmdFrntVal : Inport  Port=15
  MotTqCmdRearVal : Inport  Port=16
  PedDep : Inport  Port=17
  SAS_AnglVal : Inport  Port=18
  BrkPed : Inport  Port=19
  State : Inport  Port=20
  MotCoastFrntTq : Inport  Port=21
  MotCoastRearTq : Inport  Port=22
  H_FL : Inport  Port=23
  H_FR : Inport  Port=24
  H_RL : Inport  Port=25
  H_RR : Inport  Port=26
  Abs1 : Abs  Commented=on  OutDataTypeStr=single  SaturateOnIntegerOverflow=off
  Abs2 : Abs  Commented=on  SaturateOnIntegerOverflow=off  OutDataTypeStr=Inherit: Inherit via internal rule
  Abs4 : Abs  OutDataTypeStr=single  SaturateOnIntegerOverflow=off
  Add10 : Sum  OutDataTypeStr=single
  Add11 : Sum  Inputs=+-  OutDataTypeStr=single
  Add12 : Sum  Inputs=+-  OutDataTypeStr=single
  Add16 : Sum  Commented=on  Inputs=+-  OutDataTypeStr=single
  Add3 : Sum  OutDataTypeStr=single
  Add7 : Sum  Commented=on  Inputs=+-
  Add9 : Sum  Inputs=+--  OutDataTypeStr=single
  Chart : Stateflow chart  TreatAsAtomicUnit=on
      settings: PortSchema="{\"entries\":[{\"content\":{\"sides\":[{\"content\":{\"connectorIds\":[\"In1\",\"In2\",\"In3\",\"In4\",\"In5\",\"In6\",\"In7\",\"In9\",\"In8\",\"In10\",\"In11\",\"In12\"]},\"type\":\"ConnectorPlacement.EquallySpacedRectSide\",\"uuid\":\"75b2ab73-8438-4a11-8d44-3c554863d251\"},{\"content\":{\"connectorIds\":[\"Out1\"],\"side\":\"RIGHT\"},\"type\":\"ConnectorPlacement.EquallySpacedRectSide\",\"uuid\":\"5aeb794d-9c2f-4121-b9ec-3eb8d952f635\"},{\"content\":{\"side\":\"TOP\"},\"type\":\"ConnectorPlacement.EquallySpacedRectSide\",\"uuid\":\"df0c7b2f-a7fc-4cdf-b14b-b147e9110bf4\"}]},\"type\":\"ConnectorPlacement.EquallySpacedConnector\",\"uuid\":\"e5effcba-59ca-4619-a453-6d90fda198a7\"}],\"packageUris\":[\"http://schema.mathworks.com/mf0/Connector/R2020b\"],\"version\":\"1.0\"}"
  Compare To Constant{,1,4,6} (4 alike) : simulink/Logic and Bit Operations/Compare To Constant  relop=>=  const=2  OutDataTypeStr=boolean
  Compare To Constant{2..3,5,7} (4 alike) : simulink/Logic and Bit Operations/Compare To Constant  relop=~=  const=0  OutDataTypeStr=boolean
  Constant{,1,5..6} (4 alike) : Constant  Value=switch_logic
  Constant{10..13} (4 alike) : Constant  Value=VmcRgn_slip_max_C  OutDataTypeStr=single
  Constant14 : Constant  Commented=on  Value=0  OutDataTypeStr=single
  Constant2 : Constant  Commented=on
  Constant25 : Constant  Value=VmcRgn_Yaw_thrs_C  OutDataTypeStr=single
  Constant26 : Constant  Value=VmcRgn_PedDep_thrs_C  OutDataTypeStr=single
  Constant27 : Constant  Value=VmcRgn_SAS_thrs_C  OutDataTypeStr=single
  Constant3 : Constant  Commented=on  Value=0
  Constant4 : Constant  Value=VmcRgn_r_e_C
  Constant7 : Constant  Commented=on  OutDataTypeStr=single
  Constant8 : Constant  Value=VmcRgn_J_C
  Constant9 : Constant  Value=VmcRgn_target_w_acc_C
  Delay One Step{,1..2,4} (4 alike) : Delay  DelayLength=1
  Delay{1..10} (10 alike) : Delay  DelayLength=1
  Demux2 : Demux
  Divide : Product  Inputs=*/
  Equal{,1..3} (4 alike) : RelationalOperator  Operator===  OutDataTypeStr=boolean  RndMeth=Simplest  InputSameDT=off
  From12 : From  Commented=on  GotoTag=rd_r
  From{36,38,56,58} (4 alike) : From  Commented=on  GotoTag=DesYawRtVal
  From{37,39,57,61} (4 alike) : From  Commented=on  GotoTag=IMU_YawRtVal
  From6 : From  Commented=on  GotoTag=rd_r
  Gain4 : Gain  Gain=VmcRgn_slip_max_gain_F_C  OutDataTypeStr=single
  Gain5 : Gain  Gain=VmcRgn_slip_max_gain_F_C  OutDataTypeStr=single
  Gain6 : Gain  Gain=VmcRgn_slip_max_gain_R_C  OutDataTypeStr=single
  Gain7 : Gain  Gain=VmcRgn_slip_max_gain_R_C  OutDataTypeStr=single
  Goto2 : Goto  Commented=on  GotoTag=yaw_flag
  Goto27 : Goto  Commented=on  GotoTag=yaw_flag
  Goto28 : Goto  Commented=on  GotoTag=rd_r
  Goto8 : Goto  Commented=on  GotoTag=rd_r
  Logical Operator{1..5,12..16} (10 alike) : Logic  Operator=OR  AllPortsSameDT=off  OutDataTypeStr=boolean
  Max2 : MinMax  Function=max  Inputs=2  OutDataTypeStr=single
  Max3 : MinMax  Function=max  Inputs=2  OutDataTypeStr=single
  Mux : Mux  Inputs=2
  Mux1 : Mux
  Mux12 : Mux
  Mux2 : Mux  Inputs=2
  Product10 : Product  OutDataTypeStr=single
  Product9 : Product  OutDataTypeStr=single
  Relational Operator{5..8} (4 alike) : RelationalOperator  Operator=<  OutDataTypeStr=boolean  RndMeth=Simplest  InputSameDT=off
  Saturation2 : Saturate  UpperLimit=0  LowerLimit=-1000
  Saturation3 : Saturate  UpperLimit=5  LowerLimit=-5
  Saturation4 : Saturate  UpperLimit=0  LowerLimit=-1000  OutDataTypeStr=single
  Saturation5 : Saturate  UpperLimit=0  LowerLimit=-1000  OutDataTypeStr=single
  Saturation6 : Saturate  UpperLimit=0  LowerLimit=-1000
  Saturation7 : Saturate  UpperLimit=5  LowerLimit=-5
  Scope : Scope  Commented=on
  Scope{1,4,6,16} (4 alike) : Scope  NumInputPorts=2
  Scope12 : Scope  NumInputPorts=4
  Scope13 : Scope  NumInputPorts=4
  Scope{5,8..9,14} (4 alike) : Scope  Commented=on  NumInputPorts=2
  Scope{2,15,19..21} (5 alike) : Scope
  Scope22 : Scope  NumInputPorts=3
  Scope3 : Scope  Commented=on
  Scope7 : Scope  Commented=on
  Subtract : Sum  Inputs=+-
  Subtract1 : Sum  Inputs=+-
  Switch : Switch  Commented=on  Criteria=u2 > Threshold  Threshold=0.05  OutDataTypeStr=single  SaturateOnIntegerOverflow=off  InputSameDT=off
  Switch{1,3..5} (4 alike) : Switch  Criteria=u2 > Threshold  SaturateOnIntegerOverflow=off  InputSameDT=off
  Switch2 : Switch  Commented=on  Criteria=u2 > Threshold  Threshold=yaw_flag  OutDataTypeStr=single  SaturateOnIntegerOverflow=off  InputSameDT=off
  Switch{6..9} (4 alike) : Switch  Criteria=u2 > Threshold  Threshold=1  SaturateOnIntegerOverflow=off  InputSameDT=off
  Triggered Subsystem2 : Subsystem  TreatAsAtomicUnit=on
  Triggered Subsystem3 : Subsystem  TreatAsAtomicUnit=on
  Triggered Subsystem6 : Subsystem  TreatAsAtomicUnit=on
  Triggered Subsystem9 : Subsystem  TreatAsAtomicUnit=on
  yaw_flag : Outport
  Tr_regen_2 : Outport  Port=2
  Tf_regen_3 : Outport  Port=3
  Tb_max_F : Outport  Port=4
  Tb_max_R : Outport  Port=5
  H_F : Outport  Port=6
  H_R : Outport  Port=7
  Tf_regen : Outport  Port=8
  Tr_regen : Outport  Port=9
  wires:
  From38/1 -> Scope8/1
  From39/1 -> Scope8/2
  From36/1 -> Add7/1
  From37/1 -> Add7/2
  Abs2/1 -> Scope5/1, Goto8/1
  From12/1 -> Switch/2
  Constant2/1 -> Switch/1
  Constant3/1 -> Switch/3
  [TireForce_FL] -> Scope12/1, Mux12/1
  [TireForce_FR] -> Scope12/2, Mux12/2
  [TireForce_RL] -> Scope12/3, Mux12/3
  [TireForce_RR] -> Scope12/4, Mux12/4
  Mux12/1 -> Product9/2
  Constant4/1 -> Product9/1
  Constant8/1 -> Product10/1
  Constant9/1 -> Product10/2
  Product9/1 -> Add11/1
  Product10/1 -> Add11/2
  Add11/1 -> Divide/1
  Demux2/1 -> Scope13/1, [Tb_max_FL]
  Demux2/2 -> Scope13/2, [Tb_max_FR]
  Demux2/3 -> Scope13/3, [Tb_max_RL]
  Demux2/4 -> Scope13/4, [Tb_max_RR]
  Switch/1 -> Scope14/1, Scope/1, Goto2/1
  DesYawRtVal/1 -> [DesYawRtVal]
  IMU_YawRtVal/1 -> [IMU_YawRtVal]
  regen_cmd_tq/1 -> [regen_cmd_tq]
  TireForce_FL/1 -> [TireForce_FL]
  TireForce_FR/1 -> [TireForce_FR]
  TireForce_RL/1 -> [TireForce_RL]
  TireForce_RR/1 -> [TireForce_RR]
  slip_pred_FL/1 -> [slip_pred_FL]
  slip_pred_FR/1 -> [slip_pred_FR]
  slip_pred_RL/1 -> [slip_pred_RL]
  slip_pred_RR/1 -> [slip_pred_RR]
  mot2whl/1 -> [mot2whl]
  [yaw_flag] -> yaw_flag/1
  [Tr_regen_2] -> Tr_regen_2/1
  [Tf_regen_3] -> Tf_regen_3/1
  [Tb_max_F_H] -> Switch6/3
  [Tf_regen] -> Tf_regen/1
  [Tr_regen] -> Tr_regen/1
  SlipCtrlFrntTq/1 -> [SlipCtrlFrntTq]
  SlipCtrlRearTq/1 -> [SlipCtrlRearTq]
  MotTqCmdFrntVal/1 -> [MotTqCmdFrntVal]
  MotTqCmdRearVal/1 -> [MotTqCmdRearVal]
  [mot2whl] -> Divide/2
  Divide/1 -> Demux2/1
  Gain7/1 -> Relational Operator8/1
  [Tb_max_FL] -> Max2/1
  Gain4/1 -> Relational Operator5/1
  Constant13/1 -> Gain7/1
  [slip_pred_FL] -> Relational Operator5/2
  [Tb_max_F] -> Triggered Subsystem9/1(In1)
  Relational Operator8/1 -> [H_RR]
  [slip_pred_RL] -> Relational Operator7/2
  Relational Operator6/1 -> [H_FR]
  Constant12/1 -> Gain6/1
  Relational Operator5/1 -> [H_FL]
  Relational Operator7/1 -> [H_RL]
  Saturation4/1 -> [Tb_max_R_H], Scope1/2
  Gain6/1 -> Relational Operator7/1
  [H_FL] -> Logical Operator5/1
  Max3/1 -> Scope6/2, [Tb_max_R]
  Gain5/1 -> Relational Operator6/1
  [Tb_max_R] -> Triggered Subsystem6/1(In1)
  [slip_pred_RR] -> Relational Operator8/2
  Saturation5/1 -> Scope1/1, [Tb_max_F_H]
  [slip_pred_FR] -> Relational Operator6/2
  Logical Operator5/1 -> Triggered Subsystem9/Trigger
  [H_RL] -> Logical Operator4/1
  [Tb_max_FR] -> Max2/2
  [Tb_max_RR] -> Max3/2
  Logical Operator4/1 -> Triggered Subsystem6/Trigger
  Constant11/1 -> Gain5/1
  [Tb_max_RL] -> Max3/1
  [H_RR] -> Logical Operator4/2
  [H_FR] -> Logical Operator5/2
  Max2/1 -> Scope6/1, [Tb_max_F]
  Constant10/1 -> Gain4/1
  Add16/1 -> Abs1/1
  From6/1 -> Switch2/2
  From61/1 -> Scope9/2
  From58/1 -> Scope9/1
  Switch2/1 -> Scope14/2, Goto27/1, Scope3/1
  From57/1 -> Add16/2
  From56/1 -> Add16/1
  Constant14/1 -> Switch2/3
  Constant7/1 -> Switch2/1
  Abs1/1 -> Scope7/1, Scope5/2, Goto28/1
  PedDep/1 -> [PedDep]
  SAS_AnglVal/1 -> [SAS_AnglVal]
  Constant25/1 -> Chart/6(Yawthrs)
  Constant26/1 -> Chart/4(PedDepthrs)
  Constant27/1 -> Chart/5(SASthrs)
  [SAS_AnglVal] -> Chart/3(SASAngle)
  [PedDep] -> Chart/2(PedDep)
  Add12/1 -> Abs4/1
  [DesYawRtVal] -> Add12/1
  [IMU_YawRtVal] -> Add12/2
  Abs4/1 -> Chart/1(rd_r)
  BrkPed/1 -> [BrkPed]
  [BrkPed] -> Chart/7(BrkPed)
  Add7/1 -> Abs2/1
  [H_F] -> Scope16/1
  [H_R] -> Scope16/2
  State/1 -> [State]
  [State] -> Compare To Constant/1
  Compare To Constant/1 -> Logical Operator2/1
  [yaw_flag] -> Compare To Constant2/1
  Compare To Constant2/1 -> Logical Operator2/2
  [H_FR] -> Logical Operator1/2
  [H_FL] -> Logical Operator1/1
  Logical Operator1/1 -> Switch3/1, Equal/1
  Logical Operator2/1 -> Equal/2
  Equal/1 -> Switch3/2
  Switch3/1 -> Delay6/1, [H_F]
  Delay6/1 -> Switch3/3
  [yaw_flag] -> Compare To Constant3/1
  Switch4/1 -> Delay7/1, [H_R]
  Logical Operator12/1 -> Equal1/2
  [State] -> Compare To Constant1/1
  Logical Operator3/1 -> Switch4/1, Equal1/1
  Compare To Constant3/1 -> Logical Operator12/2
  [H_RL] -> Logical Operator3/1
  Delay7/1 -> Switch4/3
  Compare To Constant1/1 -> Logical Operator12/1
  [H_RR] -> Logical Operator3/2
  Equal1/1 -> Switch4/2
  Triggered Subsystem9/1(Out1) -> Saturation5/1
  Triggered Subsystem6/1(Out1) -> Saturation4/1
  [MotTqCmdFrntVal] -> Delay8/1
  [MotTqCmdRearVal] -> Delay9/1
  MotCoastFrntTq/1 -> [MotCoastFrntTq]
  MotCoastRearTq/1 -> [MotCoastRearTq]
  [MotCoastFrntTq] -> Chart/10(MotCoastFrntTq)
  [MotCoastRearTq] -> Chart/11(MotCoastRearTq)
  Delay8/1 -> Chart/9(MotTqCmdFrntVal)
  Delay9/1 -> Chart/8(MotTqCmdRearVal)
  [State] -> Chart/12(state)
  Chart/1(YawFlag) -> Scope2/1, [yaw_flag]
  [regen_cmd_tq] -> Add9/1
  [MotTqCmdFrntVal] -> Delay2/1
  [MotTqCmdRearVal] -> Delay3/1
  Add9/1 -> Scope21/1, [tq_give]
  [tq_give] -> Saturation3/1
  Saturation3/1 -> Add10/1, Scope20/1
  Delay10/1 -> Add10/2
  Saturation6/1 -> Scope19/1, [Tr_regen_2]
  Add10/1 -> Saturation6/1
  [MotTqCmdRearVal] -> Delay10/1
  Add3/1 -> Saturation2/1
  Delay1/1 -> Add3/2
  Saturation2/1 -> Scope15/1, [Tf_regen_3]
  Saturation7/1 -> Add3/1
  [tq_give] -> Saturation7/1
  [MotTqCmdFrntVal] -> Delay1/1
  Delay2/1 -> Add9/2
  Delay3/1 -> Add9/3
  [H_F_] -> Triggered Subsystem2/Trigger
  Switch1/1 -> [H_F_], Delay One Step2/1
  Logical Operator13/1 -> Switch1/1, Equal2/1
  Equal2/1 -> Switch1/2
  [MotTqCmdFrntVal] -> Delay One Step/1
  [H_FL_] -> Logical Operator13/1
  [H_FR_] -> Logical Operator13/2
  Delay One Step2/1 -> Switch1/3
  Triggered Subsystem2/1(Out1) -> [Tb_max_F_H_]
  Logical Operator15/1 -> Equal3/2
  [H_R_] -> Triggered Subsystem3/Trigger
  Switch5/1 -> [H_R_], Delay One Step1/1
  Logical Operator14/1 -> Switch5/1, Equal3/1
  Equal3/1 -> Switch5/2
  [MotTqCmdRearVal] -> Delay One Step4/1
  [H_RL_] -> Logical Operator14/1
  [H_RR_] -> Logical Operator14/2
  Delay One Step1/1 -> Switch5/3
  Triggered Subsystem3/1(Out1) -> [Tb_max_R_H_]
  [State] -> Compare To Constant4/1
  Compare To Constant4/1 -> Logical Operator15/1
  [yaw_flag] -> Compare To Constant5/1
  Compare To Constant5/1 -> Logical Operator15/2
  Logical Operator16/1 -> Equal2/2
  [State] -> Compare To Constant6/1
  [yaw_flag] -> Compare To Constant7/1
  Compare To Constant6/1 -> Logical Operator16/1
  Compare To Constant7/1 -> Logical Operator16/2
  Delay One Step/1 -> Triggered Subsystem2/1(In1)
  Delay One Step4/1 -> Triggered Subsystem3/1(In1)
  H_FL/1 -> [H_FL_]
  H_FR/1 -> [H_FR_]
  H_RL/1 -> [H_RL_]
  H_RR/1 -> [H_RR_]
  Constant/1 -> Switch6/2
  Switch6/1 -> Tb_max_F/1
  [Tb_max_F_H_] -> Switch6/1
  [Tb_max_R_H_] -> Switch7/1
  Constant1/1 -> Switch7/2
  [Tb_max_R_H] -> Switch7/3
  Switch7/1 -> Tb_max_R/1
  Constant5/1 -> Switch8/2
  [H_F] -> Switch8/3
  Switch8/1 -> H_F/1
  [H_F_] -> Switch8/1
  Switch9/1 -> H_R/1
  [H_R] -> Switch9/3
  [H_R_] -> Switch9/1
  Constant6/1 -> Switch9/2
  [Tb_max_F] -> Mux/1
  [H_R] -> Mux2/2
  [TireForce_RL] -> Mux1/3
  [Tb_max_R] -> Mux/2
  [H_F] -> Mux2/1
  [TireForce_FL] -> Mux1/1
  Mux1/1 -> Scope22/1
  [TireForce_FR] -> Mux1/2
  Mux2/1 -> Scope22/3
  Mux/1 -> Scope22/2
  [TireForce_RR] -> Mux1/4
  ? -> ?
  ? -> ?
  [MotTqCmdRearVal] -> Delay5/1
  [MotCoastFrntTq] -> Subtract/2
  [MotTqCmdFrntVal] -> Delay4/1
  [MotCoastRearTq] -> Subtract1/2
  Delay4/1 -> Subtract/1
  Delay5/1 -> Subtract1/1
  Subtract/1 -> Scope4/1
  Subtract1/1 -> Scope4/2

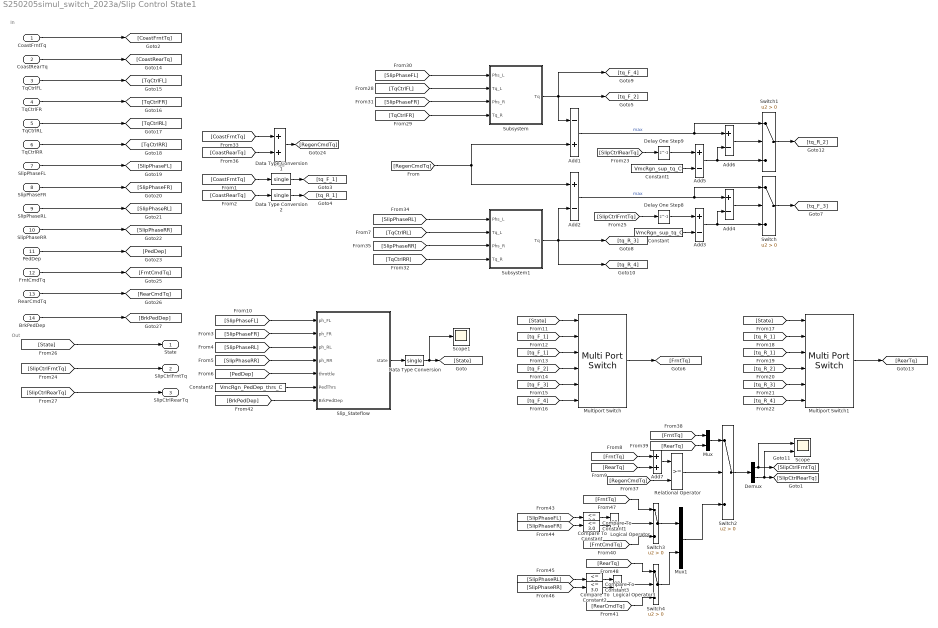
== system S250205simul_switch_2023a/Slip Control State1 ==
  note: Out
  note: In
  CoastFrntTq : Inport
  CoastRearTq : Inport  Port=2
  TqCtrlFL : Inport  Port=3
  TqCtrlFR : Inport  Port=4
  TqCtrlRL : Inport  Port=5  LockScale=on
  TqCtrlRR : Inport  Port=6
  SlipPhaseFL : Inport  Port=7
  SlipPhaseFR : Inport  Port=8
  SlipPhaseRL : Inport  Port=9
  SlipPhaseRR : Inport  Port=10
  PedDep : Inport  Port=11
  FrntCmdTq : Inport  Port=12
  RearCmdTq : Inport  Port=13
  BrkPedDep : Inport  Port=14
  Add : Sum
  Add1 : Sum  Inputs=-+
  Add{2..6} (5 alike) : Sum  Inputs=+-
  Add7 : Sum
  Compare To Constant{,1..3} (4 alike) : simulink/Logic and Bit Operations/Compare To Constant  relop=<=  const=3.0  OutDataTypeStr=boolean
  Constant : Constant  Value=VmcRgn_sup_tq_C  OutDataTypeStr=single
  Constant1 : Constant  Value=VmcRgn_sup_tq_C  OutDataTypeStr=single
  Constant2 : Constant  Value=VmcRgn_PedDep_thrs_C
  Data Type Conversion : DataTypeConversion  OutDataTypeStr=single  SaturateOnIntegerOverflow=off  RndMeth=Floor
  Data Type Conversion1 : DataTypeConversion  OutDataTypeStr=single  SaturateOnIntegerOverflow=off  RndMeth=Floor
  Data Type Conversion2 : DataTypeConversion  OutDataTypeStr=single  SaturateOnIntegerOverflow=off  RndMeth=Floor
  Delay One Step8 : Delay  DelayLength=1
  Delay One Step9 : Delay  DelayLength=1
  Demux : Demux  Outputs=2
  Logical Operator : Logic  Operator=OR  AllPortsSameDT=off  OutDataTypeStr=boolean
  Logical Operator1 : Logic  Operator=OR  AllPortsSameDT=off  OutDataTypeStr=boolean
  Multiport Switch : MultiPortSwitch  DataPortOrder=Zero-based contiguous  Inputs=5  zeroidx=on  SaturateOnIntegerOverflow=off  InputSameDT=off
  Multiport Switch1 : MultiPortSwitch  DataPortOrder=Zero-based contiguous  Inputs=5  zeroidx=on  SaturateOnIntegerOverflow=off  InputSameDT=off
  Mux : Mux  Inputs=2
  Mux1 : Mux  Inputs=2
  Relational Operator : RelationalOperator  OutDataTypeStr=boolean  RndMeth=Simplest  InputSameDT=off
  Scope : Scope  NumInputPorts=2
  Scope1 : Scope
  Slip_Stateflow : Stateflow chart  TreatAsAtomicUnit=on
  Subsystem : Subsystem
  Subsystem1 : Subsystem
  Switch{,1..4} (5 alike) : Switch  Criteria=u2 > Threshold  SaturateOnIntegerOverflow=off  InputSameDT=off
  State : Outport
  SlipCtrlFrntTq : Outport  Port=2
  SlipCtrlRearTq : Outport  Port=3
  wires:
  [RegenCmdTq] -> Add1/2, Add2/1
  Add2/1 -> Switch/1, Add4/1  "max"
  [SlipCtrlRearTq] -> Delay One Step9/1
  [PedDep] -> Slip_Stateflow/5(throttle)
  Add5/1 -> Add6/2, Switch1/3
  Constant/1 -> Add3/2
  Add3/1 -> Add4/2, Switch/3
  [SlipPhaseRL] -> Slip_Stateflow/3(ph_RL)
  Add4/1 -> Switch/2
  [SlipPhaseFR] -> Slip_Stateflow/2(ph_FR)
  Constant1/1 -> Add5/2
  Add1/1 -> Switch1/1, Add6/1  "max"
  Delay One Step8/1 -> Add3/1
  Switch1/1 -> [tq_R_2]
  Switch/1 -> [tq_F_3]
  Subsystem1/1(Tq) -> Add2/2, [tq_R_4], [tq_R_3]
  [SlipPhaseRR] -> Slip_Stateflow/4(ph_RR)
  Add6/1 -> Switch1/2
  Slip_Stateflow/1(state) -> Data Type Conversion/1
  Delay One Step9/1 -> Add5/1
  Subsystem/1(Tq) -> Add1/1, [tq_F_2], [tq_F_4]
  [SlipPhaseFL] -> Slip_Stateflow/1(ph_FL)
  [SlipCtrlFrntTq] -> Delay One Step8/1
  Data Type Conversion/1 -> Scope1/1, [State]
  [State] -> State/1
  [SlipCtrlFrntTq] -> SlipCtrlFrntTq/1
  [SlipCtrlRearTq] -> SlipCtrlRearTq/1
  RearCmdTq/1 -> [RearCmdTq]
  CoastRearTq/1 -> [CoastRearTq]
  TqCtrlFR/1 -> [TqCtrlFR]
  TqCtrlRL/1 -> [TqCtrlRL]
  SlipPhaseFR/1 -> [SlipPhaseFR]
  TqCtrlFL/1 -> [TqCtrlFL]
  PedDep/1 -> [PedDep]
  SlipPhaseFL/1 -> [SlipPhaseFL]
  SlipPhaseRR/1 -> [SlipPhaseRR]
  SlipPhaseRL/1 -> [SlipPhaseRL]
  CoastFrntTq/1 -> [CoastFrntTq]
  TqCtrlRR/1 -> [TqCtrlRR]
  FrntCmdTq/1 -> [FrntCmdTq]
  [SlipPhaseFR] -> Subsystem/3(Phs_R)
  [SlipPhaseFL] -> Subsystem/1(Phs_L)
  [TqCtrlFL] -> Subsystem/2(Tq_L)
  [TqCtrlFR] -> Subsystem/4(Tq_R)
  Data Type Conversion2/1 -> [tq_R_1]
  [CoastFrntTq] -> Add/1
  [CoastRearTq] -> Data Type Conversion2/1
  [CoastFrntTq] -> Data Type Conversion1/1
  [CoastRearTq] -> Add/2
  Add/1 -> [RegenCmdTq]
  Data Type Conversion1/1 -> [tq_F_1]
  [TqCtrlRR] -> Subsystem1/4(Tq_R)
  [TqCtrlRL] -> Subsystem1/2(Tq_L)
  [SlipPhaseRL] -> Subsystem1/1(Phs_L)
  [SlipPhaseRR] -> Subsystem1/3(Phs_R)
  Demux/1 -> Scope/1, [SlipCtrlFrntTq]
  [RegenCmdTq] -> Relational Operator/2
  Switch2/1 -> Demux/1
  Relational Operator/1 -> Switch2/2
  Multiport Switch1/1 -> [RearTq]
  Add7/1 -> Relational Operator/1
  [FrntTq] -> Mux/1
  Mux1/1 -> Switch2/3
  [tq_R_1] -> Multiport Switch1/3
  [RearTq] -> Add7/2
  [FrntTq] -> Add7/1
  [tq_R_2] -> Multiport Switch1/4
  [tq_F_3] -> Multiport Switch/5
  [RearTq] -> Mux/2
  [tq_F_4] -> Multiport Switch/6
  Multiport Switch/1 -> [FrntTq]
  [tq_R_3] -> Multiport Switch1/5
  Mux/1 -> Switch2/1
  [tq_F_1] -> Multiport Switch/2
  Demux/2 -> Scope/2, [SlipCtrlRearTq]
  [tq_F_1] -> Multiport Switch/3
  [tq_F_2] -> Multiport Switch/4
  [State] -> Multiport Switch1/1
  [State] -> Multiport Switch/1
  [tq_R_4] -> Multiport Switch1/6
  [tq_R_1] -> Multiport Switch1/2
  Constant2/1 -> Slip_Stateflow/6(PedThrs)
  BrkPedDep/1 -> [BrkPedDep]
  [BrkPedDep] -> Slip_Stateflow/7(BrkPedDep)
  Switch3/1 -> Mux1/1
  [FrntCmdTq] -> Switch3/3
  [FrntTq] -> Switch3/1
  [SlipPhaseFL] -> Compare To Constant/1
  [SlipPhaseFR] -> Compare To Constant1/1
  Compare To Constant/1 -> Logical Operator/1
  Compare To Constant1/1 -> Logical Operator/2
  Logical Operator/1 -> Switch3/2
  Switch4/1 -> Mux1/2
  Compare To Constant3/1 -> Logical Operator1/2
  Compare To Constant2/1 -> Logical Operator1/1
  Logical Operator1/1 -> Switch4/2
  [SlipPhaseRR] -> Compare To Constant3/1
  [SlipPhaseRL] -> Compare To Constant2/1
  [RearCmdTq] -> Switch4/3
  [RearTq] -> Switch4/1
